simulink model "QAM_modelo"  (R2020b)
settings: Solver=VariableStepAuto  StartTime=0.0  StopTime=203*6  MaxStep=1e-3  MinStep=1e-4  RelTol=1e-3
values from neighbouring files (symbols this model uses):
  Pd = 40    [simulacion_qam.m]    (also in simulacioon.m)
libraries: commdigbbndam3 x2
settings Model: Creator=Mateo  LastModifiedBy=Mateo
settings SolverCC: InitialStep=1e-3
settings DataIOCC: ReturnWorkspaceOutputs=off

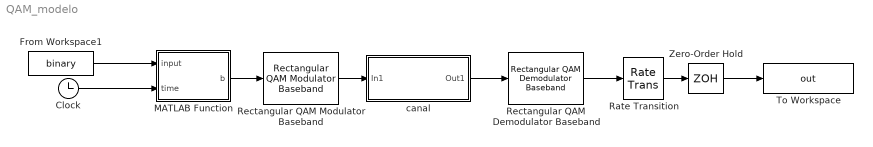
== system QAM_modelo ==
  Clock : Clock
  From Workspace1 : FromWorkspace  VariableName=binary
  MATLAB Function : MATLAB Function  TreatAsAtomicUnit=on
  Rate Transition : RateTransition
  Rectangular QAM Demodulator Baseband : commdigbbndam3/Rectangular QAM Demodulator Baseband  M=8  OutType=Integer  DecType=Hard decision  VarSource=Dialog  Variance=1  Dec=Binary  Mapping=[0:15]  PowType=Average Power  MinDist=2  AvgPow=1  PeakPow=1  Ph=0  outDtype1=Inherit via internal rule  outDtype2=Inherit via internal rule  derotateFactorWordLen=16  derotateFactorDataTypeStr=Inherit: Same word length as input  derotateFactorLastDataTypeStr=Inherit: Same word length as input  denormFactorWordLen=16  denormFactorDataTypeStr=Inherit: Same word length as input  denormFactorLastDataTypeStr=Inherit: Same word length as input  prodOutWordLen=32  prodOutOverflowMode=Wrap  prodOutRoundingMode=Floor  prodOutOvFlMode=off  prodOutOvFlModeLastStrValue=off  sumWordLen=32
  Rectangular QAM Modulator Baseband : commdigbbndam3/Rectangular QAM Modulator Baseband  M=8  InType=Integer  Enc=Binary  Mapping=[0:15]  PowType=Average Power  MinDist=2  AvgPow=1  PeakPow=1  Ph=0  outDtype=double  outWordLen=16  outUDDataType=sfix(16)  outFracLenMode=Best precision  outFracLen=15  outDataTypeStr=double  outLastDataTypeStr=double
  To Workspace : ToWorkspace  VariableName=out  SaveFormat=Timeseries  SampleTime=-1
  Zero-Order Hold : ZeroOrderHold  SampleTime=6
  canal : Subsystem
  wires:
  From Workspace1/1 -> MATLAB Function/1(input)
  Clock/1 -> MATLAB Function/2(time)
  MATLAB Function/1(b) -> Rectangular QAM Modulator Baseband/1
  Rectangular QAM Demodulator Baseband/1 -> Rate Transition/1
  Rate Transition/1 -> Zero-Order Hold/1
  Zero-Order Hold/1 -> To Workspace/1
  Rectangular QAM Modulator Baseband/1 -> canal/1(In1)
  canal/1(Out1) -> Rectangular QAM Demodulator Baseband/1

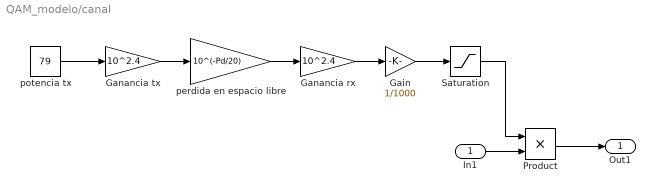
== system QAM_modelo/canal ==
  In1 : Inport
  Gain : Gain  Gain=1/1000
  Ganancia rx : Gain  Gain=10^2.4
  Ganancia tx : Gain  Gain=10^2.4
  Product : Product
  Saturation : Saturate  UpperLimit=1  LowerLimit=0
  perdida en espacio libre : Gain  Gain=10^(-Pd/20)
  potencia tx : Constant  Value=79
  Out1 : Outport
  wires:
  potencia tx/1 -> Ganancia tx/1
  Ganancia tx/1 -> perdida en espacio libre/1
  perdida en espacio libre/1 -> Ganancia rx/1
  Product/1 -> Out1/1
  Saturation/1 -> Product/1
  In1/1 -> Product/2
  Ganancia rx/1 -> Gain/1
  Gain/1 -> Saturation/1

== matlab function QAM_modelo/MATLAB Function ==
  data: input input; b output; time input
function b = fcn(input,time)
   b=input(floor(time/6)+1:floor(time/6)+3);
end
